simulink model "trafficLight"  (R2016a)
settings: Solver=FixedStepDiscrete  StartTime=0.0  StopTime=inf  RelTol=1e-3
settings Model: Creator=Eng. Aya Adel  LastModifiedBy=Eng. Aya Adel
settings OptimizationCC: DefaultParameterBehavior=Inlined  OptimizeModelRefInitCode=on  LifeSpan=1
settings DebuggingCC: UnderspecifiedInitializationDetection=Classic  MergeDetectMultiDrivingBlocksExec=none
settings ModelReferenceCC: PropagateSignalLabelsOutOfModel=off
settings RTWCC: SystemTargetFile=ert.tlc  GenCodeOnly=on  TemplateMakefile=ert_default_tmf  GenerateReport=on  IncludeHyperlinkInReport=on  LaunchReport=on  GenerateTraceInfo=on  GenerateTraceReport=on  GenerateTraceReportSl=on  GenerateTraceReportSf=on  GenerateTraceReportEml=on
settings CodeAppCC: ForceParamTrailComments=on  IgnoreCustomStorageClasses=off  OperatorAnnotations=on  SimulinkDataObjDesc=on  SFDataObjDesc=on  MATLABFcnDesc=on  InsertBlockDesc=on  MATLABSourceComments=on
settings ERTTargetCC: GenerateSampleERTMain=on  InlinedParameterPlacement=NonHierarchical  ERTCustomFileTemplate=example_file_process.tlc

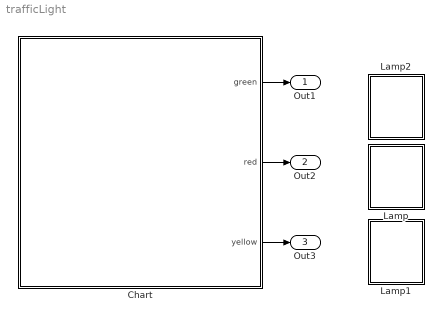
== system trafficLight ==
  Chart : Stateflow chart  TreatAsAtomicUnit=on
  Lamp : Subsystem  DialogController=hmiCreateDDGDialog  IsWebBlock=on  mask(MWDashboardBlock){webBlockId=95812472-36a1-47b4-a98e-5dcbce0202c2, webBlockType=lamp, ShowInLibBrowser=on, ShowInitialText=on, HMISrcModelName=trafficLight}
      mask prompts: webBlockType "WebBlock Type"; HMISrcModelName "Source Model"
      mask Help: helpview([docroot '/mapfiles/simulink.map'], 'hmi_lamp')
      mask Display:
      | if strcmp(get_param(bdroot(gcb),'BlockDiagramType'), 'library')
      |     image([(matlabroot) '/toolbox/simulink/hmi/icons/Lamp.png']);
      | end
  Lamp1 : Subsystem  DialogController=hmiCreateDDGDialog  IsWebBlock=on  mask(MWDashboardBlock){webBlockId=227e6077-e267-458e-a320-e56d8c87c446, webBlockType=lamp, ShowInLibBrowser=on, ShowInitialText=on, HMISrcModelName=trafficLight}
      mask prompts: webBlockType "WebBlock Type"; HMISrcModelName "Source Model"
      mask Help: helpview([docroot '/mapfiles/simulink.map'], 'hmi_lamp')
      mask Display:
      | if strcmp(get_param(bdroot(gcb),'BlockDiagramType'), 'library')
      |     image([(matlabroot) '/toolbox/simulink/hmi/icons/Lamp.png']);
      | end
  Lamp2 : Subsystem  DialogController=hmiCreateDDGDialog  IsWebBlock=on  mask(MWDashboardBlock){webBlockId=aa318a3a-6cbd-49c2-ad3c-adbb22553372, webBlockType=lamp, ShowInLibBrowser=on, ShowInitialText=on, HMISrcModelName=trafficLight}
      mask prompts: webBlockType "WebBlock Type"; HMISrcModelName "Source Model"
      mask Help: helpview([docroot '/mapfiles/simulink.map'], 'hmi_lamp')
      mask Display:
      | if strcmp(get_param(bdroot(gcb),'BlockDiagramType'), 'library')
      |     image([(matlabroot) '/toolbox/simulink/hmi/icons/Lamp.png']);
      | end
  Out1 : Outport
  Out2 : Outport  Port=2
  Out3 : Outport  Port=3
  wires:
  Chart/1(green) -> Out1/1
  Chart/2(red) -> Out2/1
  Chart/3(yellow) -> Out3/1

== system trafficLight/Lamp ==

== system trafficLight/Lamp1 ==

== system trafficLight/Lamp2 ==

== stateflow chart trafficLight/Chart ==
  state Go
    en:
    red = 0;
    green = 0;
    yellow = 0;
    du:
    red = 0;
    green = 1;
    yellow = 0;
    ex:
  state Start
    en:
    red = 0;
    green = 0;
    yellow = 0;
    du:
    red = 0;
    green = 0;
    yellow = 1;
    ex:
  state Stop
    en:
    red = 0;
    green = 0;
    yellow = 0;
    du:
    red = 1;
    green = 0;
    yellow = 0;
    ex:
  (default) -> Start
  Start -> Go : after(3000,msec)
  Stop -> Start : after(3000,msec)
  Go -> Stop : after(3000,msec)
  data: green output uint8; red output uint8; yellow output uint8
